simulink model "LMPC_sim"  (R2023b)
settings: Solver=FixedStepAuto  StartTime=0.0  StopTime=80  FixedStep=0.1  RelTol=1e-3
values from neighbouring files (symbols this model uses):
  g = 9.81    [MPCController.m]    (also in init.m = 9.8)
  m = 5    [MPCController.m]    (also in init.m)
undefined symbols (not defined in the file or in its folder): MPCController
settings Model: Creator=tonis  LastModifiedBy=mohammad
settings ModelReferenceCC: EnableRefExpFcnMdlSchedulingChecks=on

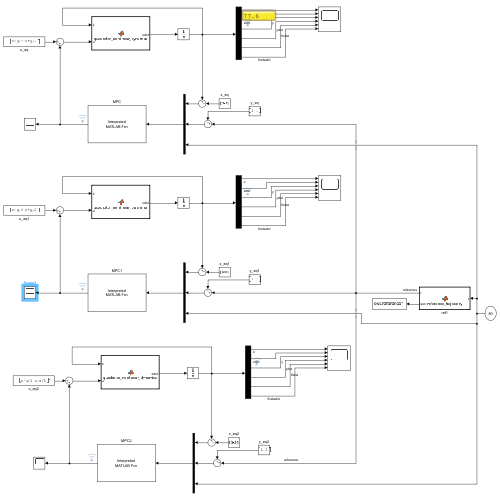
[thumbnail: Simulink's stored preview of the top-level diagram]
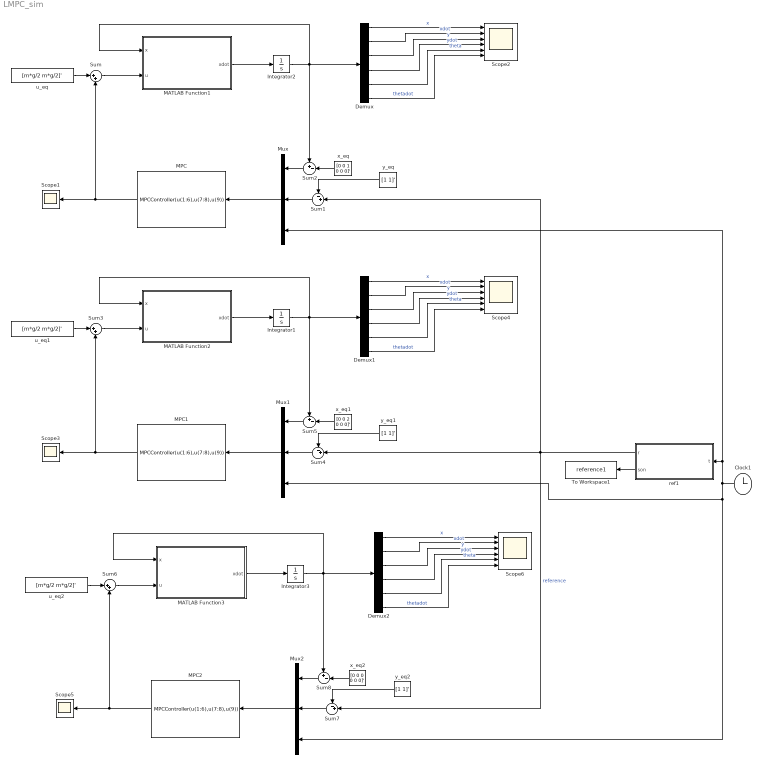
== system LMPC_sim ==
  Clock1 : Clock
  Demux : Demux  Outputs=6
  Demux1 : Demux  Outputs=6
  Demux2 : Demux  Outputs=6
  Integrator1 : Integrator  InitialCondition=[0 0 0 0 0 0]'
  Integrator2 : Integrator  InitialCondition=[0 0 0 0 0 0]'
  Integrator3 : Integrator  InitialCondition=[0 0 0 0 0 0]'
  MATLAB Function1 : MATLAB Function  TreatAsAtomicUnit=on
  MATLAB Function2 : MATLAB Function  TreatAsAtomicUnit=on
  MATLAB Function3 : MATLAB Function  TreatAsAtomicUnit=on
  MPC : MATLABFcn  MATLABFcn=MPCController(u(1:6),u(7:8),u(9))  OutputDimensions=2
  MPC1 : MATLABFcn  MATLABFcn=MPCController(u(1:6),u(7:8),u(9))  OutputDimensions=2
  MPC2 : MATLABFcn  MATLABFcn=MPCController(u(1:6),u(7:8),u(9))  OutputDimensions=2
  Mux : Mux  Inputs=3
  Mux1 : Mux  Inputs=3
  Mux2 : Mux  Inputs=3
  Scope1 : Scope
  Scope2 : Scope  NumInputPorts=6
  Scope3 : Scope
  Scope4 : Scope  NumInputPorts=6
  Scope5 : Scope
  Scope6 : Scope  NumInputPorts=6
  Sum : Sum  Inputs=|++
  Sum1 : Sum  Inputs=-+|
  Sum2 : Sum  Inputs=+-|
  Sum3 : Sum  Inputs=|++
  Sum4 : Sum  Inputs=-+|
  Sum5 : Sum  Inputs=+-|
  Sum6 : Sum  Inputs=|++
  Sum7 : Sum  Inputs=-+|
  Sum8 : Sum  Inputs=+-|
  To Workspace1 : ToWorkspace  VariableName=reference1  SaveFormat=Timeseries  SampleTime=-1
  ref1 : MATLAB Function  TreatAsAtomicUnit=on
  u_eq : Constant  Value=[m*g/2 m*g/2]'
  u_eq1 : Constant  Value=[m*g/2 m*g/2]'
  u_eq2 : Constant  Value=[m*g/2 m*g/2]'
  x_eq : Constant  Value=[0 0 1 0 0 0]'
  x_eq1 : Constant  Value=[0 0 2 0 0 0]'
  x_eq2 : Constant  Value=[0 0 0 0 0 0]'
  y_eq : Constant  Value=[1 1]'
  y_eq1 : Constant  Value=[1 1]'
  y_eq2 : Constant  Value=[1 1]'
  wires:
  MATLAB Function1/1(xdot) -> Integrator2/1
  Integrator2/1 -> Sum2/1, MATLAB Function1/1(x), Demux/1
  Demux/3 -> Scope2/3  "y"
  Demux/4 -> Scope2/4  "ydot"
  Demux/5 -> Scope2/5  "theta"
  Demux/6 -> Scope2/6  "thetadot"
  u_eq/1 -> Sum/1
  Clock1/1 -> Mux2/3, Mux1/3, Mux/3, ref1/1(t)
  Mux/1 -> MPC/1
  Sum2/1 -> Mux/1
  x_eq/1 -> Sum2/2
  Sum/1 -> MATLAB Function1/2(u)
  MPC/1 -> Scope1/1, Sum/2
  Demux/1 -> Scope2/1  "x"
  Demux/2 -> Scope2/2  "xdot"
  Sum1/1 -> Mux/2
  y_eq/1 -> Sum1/1
  MATLAB Function2/1(xdot) -> Integrator1/1
  Demux1/3 -> Scope4/3  "y"
  Demux1/5 -> Scope4/5  "theta"
  Demux1/4 -> Scope4/4  "ydot"
  Integrator1/1 -> Sum5/1, MATLAB Function2/1(x), Demux1/1
  Demux1/6 -> Scope4/6  "thetadot"
  MPC1/1 -> Scope3/1, Sum3/2
  y_eq1/1 -> Sum4/1
  ref1/2(son) -> To Workspace1/1
  Sum3/1 -> MATLAB Function2/2(u)
  Sum5/1 -> Mux1/1
  x_eq1/1 -> Sum5/2
  u_eq1/1 -> Sum3/1
  Sum4/1 -> Mux1/2
  Mux1/1 -> MPC1/1
  Demux1/2 -> Scope4/2  "xdot"
  Demux1/1 -> Scope4/1  "x"
  u_eq2/1 -> Sum6/1
  Demux2/1 -> Scope6/1  "x"
  Mux2/1 -> MPC2/1
  Sum7/1 -> Mux2/2
  Demux2/6 -> Scope6/6  "thetadot"
  ref1/1(r) -> Sum7/2, Sum4/2, Sum1/2  "reference"
  MPC2/1 -> Scope5/1, Sum6/2
  y_eq2/1 -> Sum7/1
  Sum6/1 -> MATLAB Function3/2(u)
  Sum8/1 -> Mux2/1
  Demux2/4 -> Scope6/4  "ydot"
  Integrator3/1 -> Sum8/1, MATLAB Function3/1(x), Demux2/1
  Demux2/3 -> Scope6/3  "y"
  x_eq2/1 -> Sum8/2
  Demux2/5 -> Scope6/5  "theta"
  Demux2/2 -> Scope6/2  "xdot"
  MATLAB Function3/1(xdot) -> Integrator3/1

== matlab function LMPC_sim/MATLAB Function1 ==
  data: xdot output; x input; u input

function xdot = quadrotor_nonlinear_dynamics(x, u)
% QUADROTOR_NONLINEAR_DYNAMICS Computes the nonlinear dynamics of a 2D quadrotor.
%
% Inputs:
%   t      - Time (scalar, required for ODE solvers, not used in dynamics).
%   x      - State vector [x; x_dot; y; y_dot; theta; theta_dot] (6x1).
%   u      - Input vector [u1; u2] (2x1), where u1, u2 are left/right motor thrusts.
%   params - Structure with parameters:
%            params.m - Mass of the quadrotor (kg).
%            params.g - Gravitational acceleration (m/s^2).
%            params.l - Distance from center to motors (m).
%            params.I - Moment of inertia (kg*m^2).
%
% Output:
%   xdot   - State derivative [x_dot; x_ddot; y_dot; y_ddot; theta_dot; theta_ddot] (6x1).

% Extract parameters
m = 5;
g = 9.81;
I = 1/2*m*0.25^2;

% Extract states
x1 = x(1); % x
x2 = x(2); % x_dot
x3 = x(3); % y
x4 = x(4); % y_dot
x5 = x(5); % theta
x6 = x(6); % theta_dot

% Extract inputs
u1 = u(1); % Left motor thrust
u2 = u(2); % Right motor thrust

% Compute state derivatives
xdot = zeros(6, 1);
xdot(1) = x2;                               % dx/dt = x_dot
xdot(2) = (1/m) * (u1 + u2) * sin(x5);      % d(x_dot)/dt = (u1 + u2) * sin(theta) / m
xdot(3) = x4;                               % dy/dt = y_dot
xdot(4) = (1/m) * (u1 + u2) * cos(x5) - g;  % d(y_dot)/dt = (u1 + u2) * cos(theta) / m - g
xdot(5) = x6;                               % d(theta)/dt = theta_dot
xdot(6) = (1/I) * (u1 - u2);                % d(theta_dot)/dt = l * (u1 - u2) / I

end

== matlab function LMPC_sim/MATLAB Function3 ==
  data: xdot output; x input; u input

function xdot = quadrotor_nonlinear_dynamics(x, u)
% QUADROTOR_NONLINEAR_DYNAMICS Computes the nonlinear dynamics of a 2D quadrotor.
%
% Inputs:
%   t      - Time (scalar, required for ODE solvers, not used in dynamics).
%   x      - State vector [x; x_dot; y; y_dot; theta; theta_dot] (6x1).
%   u      - Input vector [u1; u2] (2x1), where u1, u2 are left/right motor thrusts.
%   params - Structure with parameters:
%            params.m - Mass of the quadrotor (kg).
%            params.g - Gravitational acceleration (m/s^2).
%            params.l - Distance from center to motors (m).
%            params.I - Moment of inertia (kg*m^2).
%
% Output:
%   xdot   - State derivative [x_dot; x_ddot; y_dot; y_ddot; theta_dot; theta_ddot] (6x1).

% Extract parameters
m = 5;
g = 9.81;
I = 1/2*m*0.25^2;

% Extract states
x1 = x(1); % x
x2 = x(2); % x_dot
x3 = x(3); % y
x4 = x(4); % y_dot
x5 = x(5); % theta
x6 = x(6); % theta_dot

% Extract inputs
u1 = u(1); % Left motor thrust
u2 = u(2); % Right motor thrust

% Compute state derivatives
xdot = zeros(6, 1);
xdot(1) = x2;                               % dx/dt = x_dot
xdot(2) = (1/m) * (u1 + u2) * sin(x5);      % d(x_dot)/dt = (u1 + u2) * sin(theta) / m
xdot(3) = x4;                               % dy/dt = y_dot
xdot(4) = (1/m) * (u1 + u2) * cos(x5) - g;  % d(y_dot)/dt = (u1 + u2) * cos(theta) / m - g
xdot(5) = x6;                               % d(theta)/dt = theta_dot
xdot(6) = (1/I) * (u1 - u2);                % d(theta_dot)/dt = l * (u1 - u2) / I

end

== matlab function LMPC_sim/MATLAB Function2 ==
  data: xdot output; x input; u input

function xdot = quadrotor_nonlinear_dynamics(x, u)
% QUADROTOR_NONLINEAR_DYNAMICS Computes the nonlinear dynamics of a 2D quadrotor.
%
% Inputs:
%   t      - Time (scalar, required for ODE solvers, not used in dynamics).
%   x      - State vector [x; x_dot; y; y_dot; theta; theta_dot] (6x1).
%   u      - Input vector [u1; u2] (2x1), where u1, u2 are left/right motor thrusts.
%   params - Structure with parameters:
%            params.m - Mass of the quadrotor (kg).
%            params.g - Gravitational acceleration (m/s^2).
%            params.l - Distance from center to motors (m).
%            params.I - Moment of inertia (kg*m^2).
%
% Output:
%   xdot   - State derivative [x_dot; x_ddot; y_dot; y_ddot; theta_dot; theta_ddot] (6x1).

% Extract parameters
m = 5;
g = 9.81;
I = 1/2*m*0.25^2;

% Extract states
x1 = x(1); % x
x2 = x(2); % x_dot
x3 = x(3); % y
x4 = x(4); % y_dot
x5 = x(5); % theta
x6 = x(6); % theta_dot

% Extract inputs
u1 = u(1); % Left motor thrust
u2 = u(2); % Right motor thrust

% Compute state derivatives
xdot = zeros(6, 1);
xdot(1) = x2;                               % dx/dt = x_dot
xdot(2) = (1/m) * (u1 + u2) * sin(x5);      % d(x_dot)/dt = (u1 + u2) * sin(theta) / m
xdot(3) = x4;                               % dy/dt = y_dot
xdot(4) = (1/m) * (u1 + u2) * cos(x5) - g;  % d(y_dot)/dt = (u1 + u2) * cos(theta) / m - g
xdot(5) = x6;                               % d(theta)/dt = theta_dot
xdot(6) = (1/I) * (u1 - u2);                % d(theta_dot)/dt = l * (u1 - u2) / I

end

== matlab function LMPC_sim/ref1 ==
  data: r output; t input; son output
function [r, son] = reference_trajectory(t)
A = 3;
f = 0.01; % Frequency in Hz (adjust this value to change frequency)
w = 2 * pi * f;
r = [t, 10 + A * sin(w * t)]';
son = r(2);
